simulink model "PD_w_disturbance"  (R2025b)
settings: Solver=VariableStepAuto  StartTime=0.0  StopTime=2  RelTol=1e-3
settings Model: Creator=mthan  LastModifiedBy=mthan
settings SolverCC: ConsecutiveZCsStepRelTol=10*248*eps  ZeroCrossAlgorithm=Adaptive
settings DebuggingCC: IgnoredZcDiagnostic=none

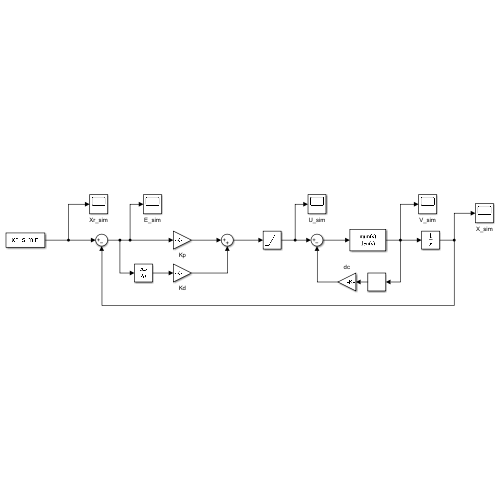
[thumbnail: Simulink's stored preview of the top-level diagram]
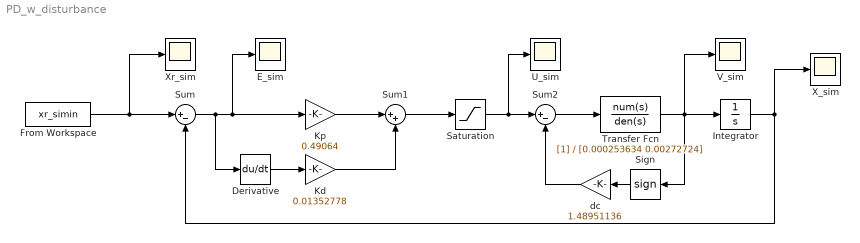
== system PD_w_disturbance ==
  Derivative : Derivative
  E_sim : Scope
      settings: ActiveDisplayYMinimum=-4.7172338627205157  ActiveDisplayYMaximum=4.7091220776127178  DataLoggingVariableName=e_sim  DataLoggingSaveFormat=Array
  From Workspace : FromWorkspace  VariableName=xr_simin  SampleTime=-1
  Integrator : Integrator
  Kd : Gain  Gain=0.01352778
  Kp : Gain  Gain=0.49064
  Saturation : Saturate  UpperLimit=10  LowerLimit=-10
  Sign : Signum
  Sum : Sum  Inputs=|+-
  Sum1 : Sum  Inputs=|++
  Sum2 : Sum  Inputs=|+-
  Transfer Fcn : TransferFcn  Denominator=[0.000253634 0.00272724]
  U_sim : Scope
      settings: ActiveDisplayYMinimum=-3.6172756028452961  ActiveDisplayYMaximum=3.6172791292282542  DataLoggingVariableName=u_sim  DataLoggingSaveFormat=Array
  V_sim : Scope
      settings: ActiveDisplayYMinimum=-1  ActiveDisplayYMaximum=1  DataLoggingVariableName=ScopeData4
  X_sim : Scope
      settings: ActiveDisplayYMinimum=-7.1389584204685352  ActiveDisplayYMaximum=56.6541529807256  DataLoggingVariableName=x_sim  DataLoggingSaveFormat=Array
  Xr_sim : Scope
      settings: ActiveDisplayYMinimum=-6.2499999999999982  ActiveDisplayYMaximum=56.25  DataLoggingVariableName=xr_sim  DataLoggingSaveFormat=Array
  dc : Gain  Gain=1.48951136
  wires:
  Derivative/1 -> Kd/1
  Sign/1 -> dc/1
  From Workspace/1 -> Sum/1, Xr_sim/1
  Sum/1 -> Derivative/1, E_sim/1, Kp/1
  Kp/1 -> Sum1/1
  Kd/1 -> Sum1/2
  Sum1/1 -> Saturation/1
  Saturation/1 -> U_sim/1, Sum2/1
  Sum2/1 -> Transfer Fcn/1
  Transfer Fcn/1 -> Sign/1, V_sim/1, Integrator/1
  Integrator/1 -> X_sim/1, Sum/2
  dc/1 -> Sum2/2
